simulink model "didier"  (R2020a)
settings: Solver=VariableStepAuto  StartTime=0.0  StopTime=50  RelTol=1e-3
values from neighbouring files (symbols this model uses):
  kd2 = eval(S.kd2)    [Lab7.m]
  kp = eval(S.kp)    [Lab7.m]
undefined symbols (not defined in the file or in its folder): kd1
settings Model: Creator=Paula  LastModifiedBy=Paula

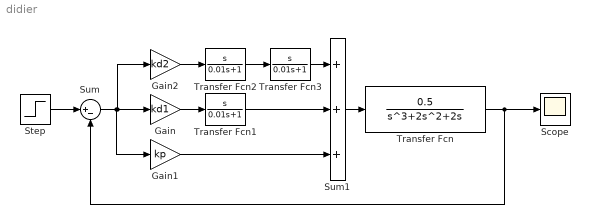
== system didier ==
  Gain : Gain  Gain=kd1
  Gain1 : Gain  Gain=kp
  Gain2 : Gain  Gain=kd2
  Scope : Scope
  Step : Step  Time=0  SampleTime=0
  Sum : Sum  Inputs=|+-
  Sum1 : Sum  Inputs=+++
  Transfer Fcn : TransferFcn  Numerator=[0.5]  Denominator=[1 2 2 0]
  Transfer Fcn1 : TransferFcn  Numerator=[1 0]  Denominator=[0.01 1]
  Transfer Fcn2 : TransferFcn  Numerator=[1 0]  Denominator=[0.01 1]
  Transfer Fcn3 : TransferFcn  Numerator=[1 0]  Denominator=[0.01 1]
  wires:
  Step/1 -> Sum/1
  Sum/1 -> Gain1/1, Gain2/1, Gain/1
  Gain/1 -> Transfer Fcn1/1
  Gain2/1 -> Transfer Fcn2/1
  Transfer Fcn1/1 -> Sum1/2
  Gain1/1 -> Sum1/3
  Sum1/1 -> Transfer Fcn/1
  Transfer Fcn/1 -> Sum/2, Scope/1
  Transfer Fcn2/1 -> Transfer Fcn3/1
  Transfer Fcn3/1 -> Sum1/1
